simulink model "course_simulink"  (R2022a)
settings: Solver=FixedStepAuto  StartTime=0.0  StopTime=0.02  RelTol=1e-3
InitFcn:
  | stop_time_as_str = get_param(gcs, 'StopTime');
  | model_stop_time = str2double(stop_time_as_str);
values from neighbouring files (symbols this model uses):
  a = [1 -3.78125206442570505 5.44829440482254412 -3.54414088511948755 0.878834866871245235]    [course_2022.m]
  amp = 3.3    [course_2022.m]
  b = [0.00319806247283222151 0 -0.00639612494566444301 0 0.00319806247283222151]    [course_2022.m]
  bias = 0    [course_2022.m]
  fraction_lenght = 18    [course_2022.m]
  freq = 650    [course_2022.m]
  word_lenght = 24    [course_2022.m]
libraries: slctrlblks x1
settings Model: DataTypeOverride=Off  MinMaxOverflowLogging=ForceOff  NumberOfSteps=10  Creator=SoloPC  LastModifiedBy=SoloPC
settings SolverCC: AlgebraicLoopSolver=TrustRegion
settings DataIOCC: SaveOutput=off  SaveTime=off
settings OptimizationCC: BlockReduction=off  ConditionallyExecuteInputs=off  DefaultParameterBehavior=Inlined
settings DebuggingCC: SignalRangeChecking=error  AlgebraicLoopMsg=error  ParameterDowncastMsg=none  ParameterOverflowMsg=none  ParameterPrecisionLossMsg=none
settings HardwareCC: ProdBitPerPointer=32  ProdBitPerSizeT=32  ProdBitPerPtrDiffT=32  ProdLargestAtomicFloat=None  ProdIntDivRoundTo=Undefined  ProdEndianess=Unspecified  ProdWordSize=32  ProdHWDeviceType=ASIC/FPGA->ASIC/FPGA  TargetBitPerPointer=64  TargetBitPerSizeT=64  TargetBitPerPtrDiffT=64  TargetLongLongMode=on  TargetIntDivRoundTo=Zero  TargetEndianess=LittleEndian  TargetWordSize=64  TargetHWDeviceType=Custom Processor->MATLAB Host Computer  ProdEqTarget=off
settings SFSimCC: CustomCodeUndefinedFunction=UseInterfaceOnly

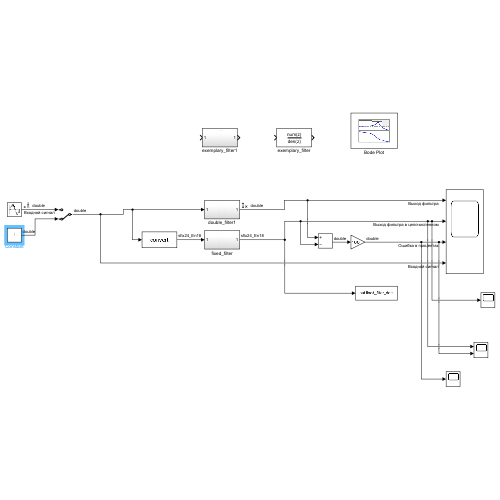
[thumbnail: Simulink's stored preview of the top-level diagram]
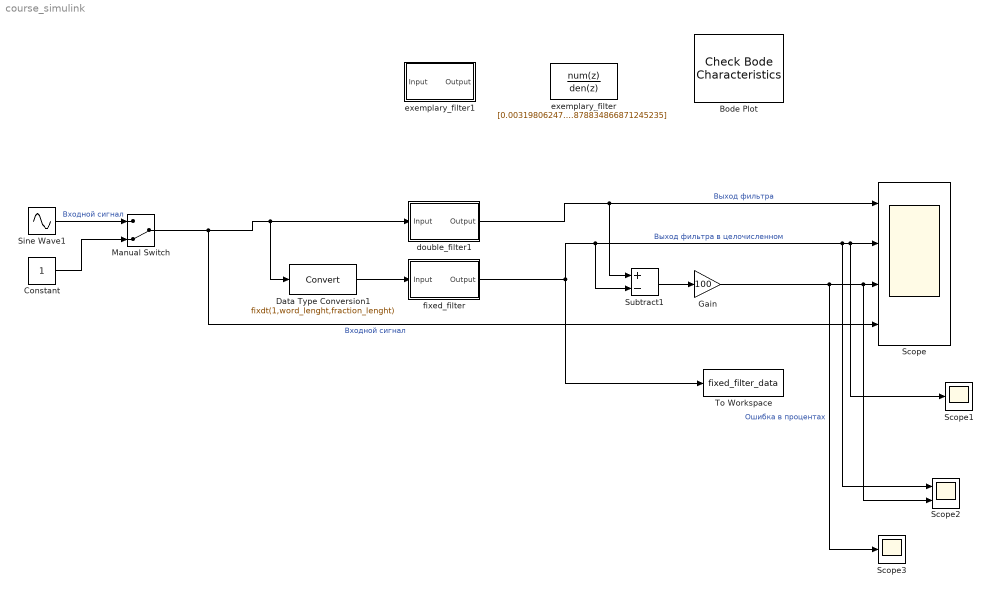
== system course_simulink ==
  Bode Plot : slctrlblks/Model Verification/Check Bode  Characteristics  InstantiateOnLoad=on  SaveOperatingPoints=off  LinearizationIOs={'/Sine Wave1', 1, 'in', 'off', '';'/double_filter1', 1, 'out', 'on', ''}  LinearizeAt=SnapshotTimes  SnapshotTimes=[0]  TriggerType=rising  SampleTime=auto  RateConversionMethod=zoh  PreWarpFreq=10  UseExactDelayModel=off  UseFullBlockNameLabels=off  UseBusSignalLabels=off  enabled=on  stopWhenAssertionFail=off  export=off  ViewDlgPos=[739 109 510 390]  OpenViewOnLoad=off  LaunchViewOnOpen=off  FrequencyUnits=rad/s  MagnitudeUnits=dB  PhaseUnits=deg  TimeUnits=seconds  EnableUpperBound=off  UpperBoundFrequencies=[]  UpperBoundMagnitudes=[]  EnableLowerBound=off  LowerBoundFrequencies=[]  LowerBoundMagnitudes=[]
  Constant : Constant
  Data Type Conversion1 : DataTypeConversion  OutDataTypeStr=fixdt(1,word_lenght,fraction_lenght)  SaturateOnIntegerOverflow=off  RndMeth=Floor
  Gain : Gain  Gain=100
  Manual Switch : ManualSwitch  CurrentSetting=0
  Scope : Scope  NumInputPorts=4
  Scope1 : Scope
  Scope2 : Scope  NumInputPorts=2
  Scope3 : Scope
  Sine Wave1 : Sin  Amplitude=amp  Bias=bias  Frequency=2 * pi * freq  SampleTime=1/16000
  Subtract1 : Sum  Inputs=+-
  To Workspace : ToWorkspace  VariableName=fixed_filter_data  SampleTime=-1
      settings: Save2DSignal=2-D array (concatenate along first dimension)
  double_filter1 : Subsystem  Tag=FilterWizardSubSystem
      settings: ErrorFcn=dspFilterRealizedInBasicElemsAlgLoopErrFcnCallback
  exemplary_filter : DiscreteFilter  Tag=BlockMethodSubSystem  Numerator=[0.00319806247283222151 0 -0.00639612494566444301 0 0.00319806247283222151]  Denominator=[1 -3.78125206442570505 5.44829440482254412 -3.54414088511948844 0.878834866871245235]  InputProcessing=Columns as channels (frame based)  FilterStructure=Direct form II transposed  a0EqualsOne=on
  exemplary_filter1 : Subsystem  Tag=FilterWizardSubSystem
      settings: ErrorFcn=dspFilterRealizedInBasicElemsAlgLoopErrFcnCallback
  fixed_filter : Subsystem  Tag=FilterWizardSubSystem
      settings: ErrorFcn=dspFilterRealizedInBasicElemsAlgLoopErrFcnCallback
  wires:
  fixed_filter/1(Output) -> To Workspace/1, Scope2/1, Scope1/1, Scope/2, Subtract1/2  "Выход фильтра в целочисленном"
  double_filter1/1(Output) -> Scope/1, Subtract1/1  "Выход фильтра"
  Data Type Conversion1/1 -> fixed_filter/1(Input)
  Subtract1/1 -> Gain/1
  Gain/1 -> Scope3/1, Scope2/2, Scope/3  "Ошибка в процентах"
  Constant/1 -> Manual Switch/2
  Sine Wave1/1 -> Manual Switch/1  "Входной сигнал"
  Manual Switch/1 -> Scope/4, double_filter1/1(Input), Data Type Conversion1/1  "Входной сигнал"

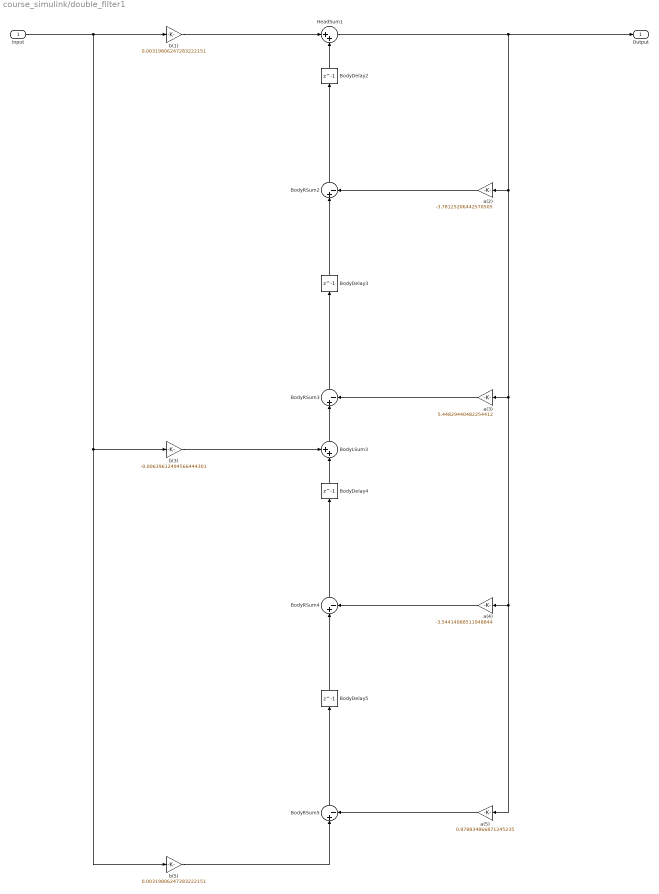
== system course_simulink/double_filter1 ==
  Input : Inport
  BodyDelay{2..5} (4 alike) : Delay  DelayLength=1  InitialCondition=0
  BodyLSum3 : Sum  Inputs=++|  RndMeth=Nearest  SaturateOnIntegerOverflow=on  OutDataTypeStr=Inherit: Same as first input
  BodyRSum{2..5} (4 alike) : Sum  Inputs=|+-  RndMeth=Nearest  SaturateOnIntegerOverflow=on  OutDataTypeStr=Inherit: Same as first input
  HeadSum1 : Sum  Inputs=|++  RndMeth=Nearest  SaturateOnIntegerOverflow=on  OutDataTypeStr=Inherit: Same as first input
  a(2) : Gain  Gain=-3.78125206442570505  ParamDataTypeStr=double  RndMeth=Nearest  SaturateOnIntegerOverflow=on  OutDataTypeStr=Inherit: Same as input
  a(3) : Gain  Gain=5.44829440482254412  ParamDataTypeStr=double  RndMeth=Nearest  SaturateOnIntegerOverflow=on  OutDataTypeStr=Inherit: Same as input
  a(4) : Gain  Gain=-3.54414088511948844  ParamDataTypeStr=double  RndMeth=Nearest  SaturateOnIntegerOverflow=on  OutDataTypeStr=Inherit: Same as input
  a(5) : Gain  Gain=0.878834866871245235  ParamDataTypeStr=double  RndMeth=Nearest  SaturateOnIntegerOverflow=on  OutDataTypeStr=Inherit: Same as input
  b(1) : Gain  Gain=0.00319806247283222151  ParamDataTypeStr=double  RndMeth=Nearest  SaturateOnIntegerOverflow=on  OutDataTypeStr=Inherit: Same as input
  b(3) : Gain  Gain=-0.00639612494566444301  ParamDataTypeStr=double  RndMeth=Nearest  SaturateOnIntegerOverflow=on  OutDataTypeStr=Inherit: Same as input
  b(5) : Gain  Gain=0.00319806247283222151  ParamDataTypeStr=double  RndMeth=Nearest  SaturateOnIntegerOverflow=on  OutDataTypeStr=Inherit: Same as input
  Output : Outport
  wires:
  Input/1 -> b(3)/1, b(5)/1, b(1)/1
  b(1)/1 -> HeadSum1/1
  HeadSum1/1 -> a(4)/1, a(5)/1, a(3)/1, a(2)/1, Output/1
  BodyRSum2/1 -> BodyDelay2/1
  a(2)/1 -> BodyRSum2/2
  BodyDelay2/1 -> HeadSum1/2
  b(3)/1 -> BodyLSum3/1
  BodyLSum3/1 -> BodyRSum3/1
  BodyRSum3/1 -> BodyDelay3/1
  a(3)/1 -> BodyRSum3/2
  BodyDelay3/1 -> BodyRSum2/1
  BodyRSum4/1 -> BodyDelay4/1
  a(4)/1 -> BodyRSum4/2
  BodyDelay4/1 -> BodyLSum3/2
  b(5)/1 -> BodyRSum5/1
  BodyRSum5/1 -> BodyDelay5/1
  a(5)/1 -> BodyRSum5/2
  BodyDelay5/1 -> BodyRSum4/1

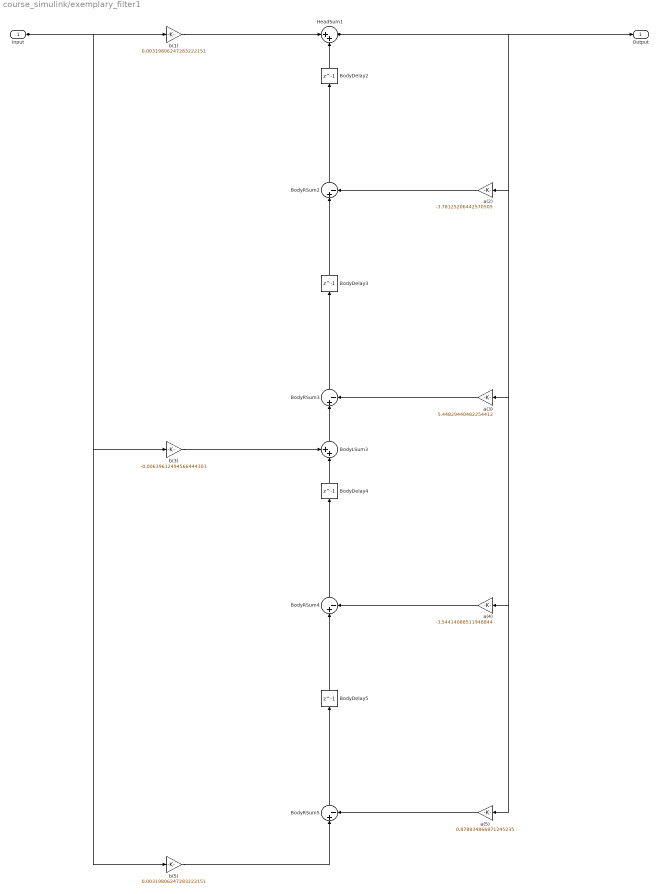
== system course_simulink/exemplary_filter1 ==
  Input : Inport
  BodyDelay{2..5} (4 alike) : Delay  DelayLength=1  InitialCondition=0
  BodyLSum3 : Sum  Inputs=++|  RndMeth=Nearest  SaturateOnIntegerOverflow=on  OutDataTypeStr=Inherit: Same as first input
  BodyRSum{2..5} (4 alike) : Sum  Inputs=|+-  RndMeth=Nearest  SaturateOnIntegerOverflow=on  OutDataTypeStr=Inherit: Same as first input
  HeadSum1 : Sum  Inputs=|++  RndMeth=Nearest  SaturateOnIntegerOverflow=on  OutDataTypeStr=Inherit: Same as first input
  a(2) : Gain  Gain=-3.78125206442570505  ParamDataTypeStr=double  RndMeth=Nearest  SaturateOnIntegerOverflow=on  OutDataTypeStr=Inherit: Same as input
  a(3) : Gain  Gain=5.44829440482254412  ParamDataTypeStr=double  RndMeth=Nearest  SaturateOnIntegerOverflow=on  OutDataTypeStr=Inherit: Same as input
  a(4) : Gain  Gain=-3.54414088511948844  ParamDataTypeStr=double  RndMeth=Nearest  SaturateOnIntegerOverflow=on  OutDataTypeStr=Inherit: Same as input
  a(5) : Gain  Gain=0.878834866871245235  ParamDataTypeStr=double  RndMeth=Nearest  SaturateOnIntegerOverflow=on  OutDataTypeStr=Inherit: Same as input
  b(1) : Gain  Gain=0.00319806247283222151  ParamDataTypeStr=double  RndMeth=Nearest  SaturateOnIntegerOverflow=on  OutDataTypeStr=Inherit: Same as input
  b(3) : Gain  Gain=-0.00639612494566444301  ParamDataTypeStr=double  RndMeth=Nearest  SaturateOnIntegerOverflow=on  OutDataTypeStr=Inherit: Same as input
  b(5) : Gain  Gain=0.00319806247283222151  ParamDataTypeStr=double  RndMeth=Nearest  SaturateOnIntegerOverflow=on  OutDataTypeStr=Inherit: Same as input
  Output : Outport
  wires:
  Input/1 -> b(1)/1, b(3)/1, b(5)/1
  b(1)/1 -> HeadSum1/1
  HeadSum1/1 -> Output/1, a(2)/1, a(3)/1, a(4)/1, a(5)/1
  BodyRSum2/1 -> BodyDelay2/1
  a(2)/1 -> BodyRSum2/2
  BodyDelay2/1 -> HeadSum1/2
  b(3)/1 -> BodyLSum3/1
  BodyLSum3/1 -> BodyRSum3/1
  BodyRSum3/1 -> BodyDelay3/1
  a(3)/1 -> BodyRSum3/2
  BodyDelay3/1 -> BodyRSum2/1
  BodyRSum4/1 -> BodyDelay4/1
  a(4)/1 -> BodyRSum4/2
  BodyDelay4/1 -> BodyLSum3/2
  b(5)/1 -> BodyRSum5/1
  BodyRSum5/1 -> BodyDelay5/1
  a(5)/1 -> BodyRSum5/2
  BodyDelay5/1 -> BodyRSum4/1

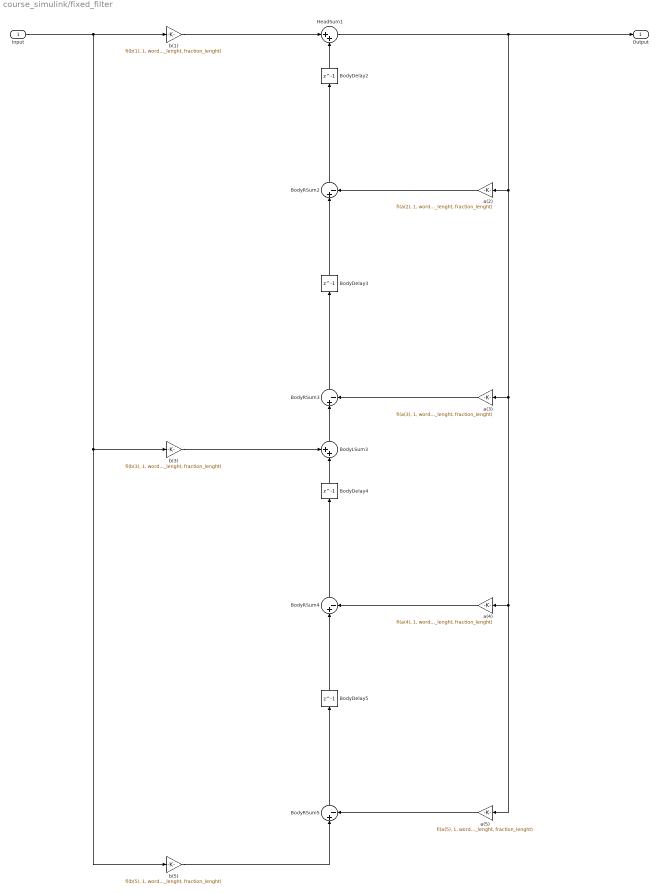
== system course_simulink/fixed_filter ==
  Input : Inport
  BodyDelay{2..5} (4 alike) : Delay  DelayLength=1  InitialCondition=0
  BodyLSum3 : Sum  Inputs=++|  SaturateOnIntegerOverflow=on  OutDataTypeStr=Inherit: Same as first input
  BodyRSum{2..5} (4 alike) : Sum  Inputs=|+-  SaturateOnIntegerOverflow=on  OutDataTypeStr=Inherit: Same as first input
  HeadSum1 : Sum  Inputs=|++  RndMeth=Nearest  SaturateOnIntegerOverflow=on  OutDataTypeStr=Inherit: Same as first input
  a(2) : Gain  Gain=fi(a(2), 1, word_lenght, fraction_lenght)  ParamDataTypeStr=double  RndMeth=Ceiling  SaturateOnIntegerOverflow=on  OutDataTypeStr=Inherit: Same as input
  a(3) : Gain  Gain=fi(a(3), 1, word_lenght, fraction_lenght)  ParamDataTypeStr=double  RndMeth=Ceiling  SaturateOnIntegerOverflow=on  OutDataTypeStr=Inherit: Same as input
  a(4) : Gain  Gain=fi(a(4), 1, word_lenght, fraction_lenght)  ParamDataTypeStr=double  RndMeth=Ceiling  SaturateOnIntegerOverflow=on  OutDataTypeStr=Inherit: Same as input
  a(5) : Gain  Gain=fi(a(5), 1, word_lenght, fraction_lenght)  ParamDataTypeStr=double  RndMeth=Ceiling  SaturateOnIntegerOverflow=on  OutDataTypeStr=Inherit: Same as input
  b(1) : Gain  Gain=fi(b(1), 1, word_lenght, fraction_lenght)  ParamDataTypeStr=double  RndMeth=Ceiling  SaturateOnIntegerOverflow=on  OutDataTypeStr=Inherit: Same as input
  b(3) : Gain  Gain=fi(b(3), 1, word_lenght, fraction_lenght)  ParamDataTypeStr=double  RndMeth=Ceiling  SaturateOnIntegerOverflow=on  OutDataTypeStr=Inherit: Same as input
  b(5) : Gain  Gain=fi(b(5), 1, word_lenght, fraction_lenght)  ParamDataTypeStr=double  RndMeth=Ceiling  SaturateOnIntegerOverflow=on  OutDataTypeStr=Inherit: Same as input
  Output : Outport
  wires:
  Input/1 -> b(3)/1, b(5)/1, b(1)/1
  HeadSum1/1 -> a(4)/1, a(5)/1, a(3)/1, a(2)/1, Output/1
  BodyRSum2/1 -> BodyDelay2/1
  a(2)/1 -> BodyRSum2/2
  BodyDelay2/1 -> HeadSum1/2
  b(3)/1 -> BodyLSum3/1
  BodyLSum3/1 -> BodyRSum3/1
  BodyRSum3/1 -> BodyDelay3/1
  a(3)/1 -> BodyRSum3/2
  BodyDelay3/1 -> BodyRSum2/1
  BodyRSum4/1 -> BodyDelay4/1
  a(4)/1 -> BodyRSum4/2
  BodyDelay4/1 -> BodyLSum3/2
  b(5)/1 -> BodyRSum5/1
  BodyRSum5/1 -> BodyDelay5/1
  a(5)/1 -> BodyRSum5/2
  BodyDelay5/1 -> BodyRSum4/1
  b(1)/1 -> HeadSum1/1
